simulink model "bipedal_robot_buV2_4"  (R2020b)
settings: Solver=ode23  StartTime=0.0  StopTime=Tsim  MaxStep=0.01  RelTol=1e-3  AbsTol=1e-3  EnableMultiTasking=on
undefined symbols (not defined in the file): Base, ctrl_config, ctrl_data, g, LefAnklePitch, LefAnkleRoll, LefHipPitch, LefHipRoll, LefHipYaw, LefKnee, lleg_str, RigAnklePitch, RigAnkleRoll, RigHipPitch, RigHipRoll, RigHipYaw, RigKnee, rleg_str, sim_floor, Tfil, TG_test_type, total_mass, Ts, X, Y, Z
libraries: sm_lib x53, biped_lib x34, nesl_utility x9, robotmaniplib x5, simulink x1, Contact_Forces_Lib x1
(part 3 of 3)

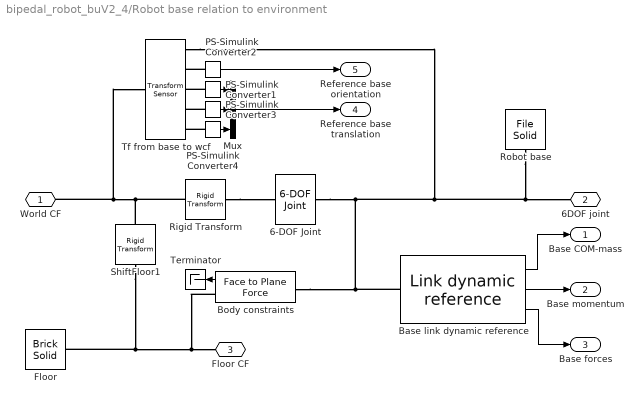
== system bipedal_robot_buV2_4/Robot base relation to environment ==
  6-DOF Joint : sm_lib/Joints/6-DOF Joint  JointMode=Normal  SenseConstraintForce=off  SenseConstraintForceX=off  SenseConstraintForceY=off  SenseConstraintForceZ=off  SenseConstraintTorque=off  SenseConstraintTorqueX=off  SenseConstraintTorqueY=off  SenseConstraintTorqueZ=off  SenseTotalForce=off  SenseTotalForceX=off  SenseTotalForceY=off  SenseTotalForceZ=off  SenseTotalTorque=off  SenseTotalTorqueX=off  SenseTotalTorqueY=off  SenseTotalTorqueZ=off  CompositeWrenchDir=FollowerOnBase  CompositeWrenchFrame=BaseFrame  PxEquilibriumPosition=0  PxEquilibriumPositionUnits=m  PxSpringStiffness=0  PxSpringStiffnessUnits=N/m  PxDampingCoefficient=0  PxDampingCoefficientUnits=N/(m/s)  PxTorqueActuationMode=NoTorque  PxMotionActuationMode=ComputedMotion  PxSensePosition=off  PxSenseVelocity=off  PxSenseAcceleration=off  PxSenseTorqueForce=off  PxSenseLowerLimitTorqueForce=off  PxSenseUpperLimitTorqueForce=off  PxLowerLimitSpecify=off  PxLowerLimitBound=-1  PxLowerLimitBoundUnits=m  PxLowerLimitStiffness=1e6  PxLowerLimitStiffnessUnits=N/m  PxLowerLimitDamping=1e3  PxLowerLimitDampingUnits=N/(m/s)  PxLowerLimitTransitionRegionWidth=1e-4  PxLowerLimitTransitionRegionWidthUnits=m  PxUpperLimitSpecify=off  PxUpperLimitBound=1  PxUpperLimitBoundUnits=m  PxUpperLimitStiffness=1e6  PxUpperLimitStiffnessUnits=N/m  PxUpperLimitDamping=1e3  PxUpperLimitDampingUnits=N/(m/s)  PxUpperLimitTransitionRegionWidth=1e-4  PxUpperLimitTransitionRegionWidthUnits=m  PxPositionTargetSpecify=on  PxPositionTargetPriority=High  PxPositionTargetValue=Base.Xinit(1)  PxPositionTargetValueUnits=m  PxVelocityTargetSpecify=off  PxVelocityTargetPriority=High  PxVelocityTargetValue=0  PxVelocityTargetValueUnits=m/s  PyEquilibriumPosition=0  PyEquilibriumPositionUnits=m  PySpringStiffness=0  PySpringStiffnessUnits=N/m  PyDampingCoefficient=0  PyDampingCoefficientUnits=N/(m/s)  PyTorqueActuationMode=NoTorque  PyMotionActuationMode=ComputedMotion  PySensePosition=off  PySenseVelocity=off  PySenseAcceleration=off  PySenseTorqueForce=off  PySenseLowerLimitTorqueForce=off  PySenseUpperLimitTorqueForce=off  PyLowerLimitSpecify=off  PyLowerLimitBound=-1  PyLowerLimitBoundUnits=m  PyLowerLimitStiffness=1e6  PyLowerLimitStiffnessUnits=N/m  PyLowerLimitDamping=1e3  PyLowerLimitDampingUnits=N/(m/s)  PyLowerLimitTransitionRegionWidth=1e-4  PyLowerLimitTransitionRegionWidthUnits=m  PyUpperLimitSpecify=off  PyUpperLimitBound=1  PyUpperLimitBoundUnits=m  PyUpperLimitStiffness=1e6  PyUpperLimitStiffnessUnits=N/m  PyUpperLimitDamping=1e3  PyUpperLimitDampingUnits=N/(m/s)  PyUpperLimitTransitionRegionWidth=1e-4  PyUpperLimitTransitionRegionWidthUnits=m  PyPositionTargetSpecify=on  PyPositionTargetPriority=High  PyPositionTargetValue=Base.Xinit(2)  PyPositionTargetValueUnits=m  PyVelocityTargetSpecify=off  PyVelocityTargetPriority=High  PyVelocityTargetValue=0  PyVelocityTargetValueUnits=m/s  PzEquilibriumPosition=0  PzEquilibriumPositionUnits=m  PzSpringStiffness=0  PzSpringStiffnessUnits=N/m  PzDampingCoefficient=0  PzDampingCoefficientUnits=N/(m/s)  PzTorqueActuationMode=NoTorque  PzMotionActuationMode=ComputedMotion  PzSensePosition=off  PzSenseVelocity=off  PzSenseAcceleration=off  PzSenseTorqueForce=off  PzSenseLowerLimitTorqueForce=off  PzSenseUpperLimitTorqueForce=off  PzLowerLimitSpecify=off  PzLowerLimitBound=0  PzLowerLimitBoundUnits=m  PzLowerLimitStiffness=1e6  PzLowerLimitStiffnessUnits=N/m  PzLowerLimitDamping=1e3  PzLowerLimitDampingUnits=N/(m/s)  PzLowerLimitTransitionRegionWidth=1e-4  PzLowerLimitTransitionRegionWidthUnits=m  PzUpperLimitSpecify=off  PzUpperLimitBound=1  PzUpperLimitBoundUnits=m  PzUpperLimitStiffness=1e6  PzUpperLimitStiffnessUnits=N/m  PzUpperLimitDamping=1e3  PzUpperLimitDampingUnits=N/(m/s)  PzUpperLimitTransitionRegionWidth=1e-4  PzUpperLimitTransitionRegionWidthUnits=m  PzPositionTargetSpecify=on  PzPositionTargetPriority=High  PzPositionTargetValue=Base.Xinit(3)  PzPositionTargetValueUnits=m  PzVelocityTargetSpecify=off  PzVelocityTargetPriority=High  PzVelocityTargetValue=0  PzVelocityTargetValueUnits=m/s  SphDefPosRotationMethod=None  SphDefPosRotationAngleUnits=deg  SphDefPosRotationStandardAxis=+Z  SphDefPosRotationAngle=0.0  SphDefPosRotationArbitraryAxis=[0 0 1]  SphDefPosFollAlignAxisA=+X  SphDefPosBaseAlignAxisA=+Y  SphDefPosFollAlignAxisB=+Y  SphDefPosBaseAlignAxisB=+Z  SphDefPosRotationSequenceAxes=FollowerAxes  SphDefPosRotationSequence=XYX  SphDefPosRotationSequenceAngles=[0 0 0]  SphDefPosRotationSequenceAnglesUnits=deg  SphDefPosRotationMatrix=[1 0 0; 0 1 0; 0 0 1]  SphEqPosRotationMethod=None  SphEqPosRotationAngleUnits=deg  SphEqPosRotationStandardAxis=+Z  SphEqPosRotationAngle=0.0  SphEqPosRotationArbitraryAxis=[0 0 1]  SphEqPosFollAlignAxisA=+X  SphEqPosBaseAlignAxisA=+Y  SphEqPosFollAlignAxisB=+Y  SphEqPosBaseAlignAxisB=+Z  SphEqPosRotationSequenceAxes=FollowerAxes  SphEqPosRotationSequence=XYX  SphEqPosRotationSequenceAngles=[0 0 0]  SphEqPosRotationSequenceAnglesUnits=deg  SphEqPosRotationMatrix=[1 0 0; 0 1 0; 0 0 1]  SphSpringStiffness=0  SphSpringStiffnessUnits=N*m/deg  SphDampingCoefficient=0  SphDampingCoefficientUnits=N*m/(deg/s)  SphActuateTorqueX=off  SphActuateTorqueY=off  SphActuateTorqueZ=off  SphActuateTorque=off  SphTorqueActuationMode=NoTorque  SphMotionActuationMode=ComputedMotion  SphActuationFrame=BaseFrame  SphSensePosition=off  SphSenseVelocityX=off  SphSenseVelocityY=off  SphSenseVelocityZ=off  SphSenseVelocity=off  SphSenseAccelerationX=off  SphSenseAccelerationY=off  SphSenseAccelerationZ=off  SphSenseAcceleration=off  SphSenseTorqueX=off  SphSenseTorqueY=off  SphSenseTorqueZ=off  SphSenseTorqueForce=off  SphSenseLowerLimitTorqueMag=off  SphSenseUpperLimitTorqueMag=off  SphSensingFrame=BaseFrame  SphLowerLimitSpecify=off  SphLowerLimitBound=15  SphLowerLimitBoundUnits=deg  SphLowerLimitStiffness=1e4  SphLowerLimitStiffnessUnits=N*m/deg  SphLowerLimitDamping=10  SphLowerLimitDampingUnits=N*m/(deg/s)  SphLowerLimitTransitionRegionWidth=0.1  SphLowerLimitTransitionRegionWidthUnits=deg  SphUpperLimitSpecify=off  SphUpperLimitBound=45  SphUpperLimitBoundUnits=deg  SphUpperLimitStiffness=1e4  SphUpperLimitStiffnessUnits=N*m/deg  SphUpperLimitDamping=10  SphUpperLimitDampingUnits=N*m/(deg/s)  SphUpperLimitTransitionRegionWidth=0.1  SphUpperLimitTransitionRegionWidthUnits=deg  SphPositionTargetRotationMethod=StandardAxis  SphPositionTargetRotationAngleUnits=rad  SphPositionTargetRotationStandardAxis=+Y  SphPositionTargetRotationAngle=0  SphPositionTargetRotationArbitraryAxis=[0 0 1]  SphPositionTargetFollAlignAxisA=+X  SphPositionTargetBaseAlignAxisA=+Y  SphPositionTargetFollAlignAxisB=+Y  SphPositionTargetBaseAlignAxisB=+Z  SphPositionTargetRotationSequenceAxes=FollowerAxes  SphPositionTargetRotationSequence=XYX  SphPositionTargetRotationSequenceAngles=[0 0 0]  SphPositionTargetRotationSequenceAnglesUnits=deg  SphPositionTargetRotationMatrix=[1 0 0; 0 1 0; 0 0 1]  SphPositionTargetSpecify=on  SphPositionTargetPriority=High  SphVelocityTargetValue=[0 0 0]  SphVelocityTargetValueUnits=deg/s  SphVelocityTargetSpecify=off  SphVelocityTargetPriority=High  SphVelocityTargetInFollowerFrame=on
  Base link dynamic reference : biped_lib/Link dynamic reference  M=Base.body.mass  I=Base.body.inertia
  Body constraints : Contact_Forces_Lib/3D/Composite Forces/Face to Plane Force  PlaB_x=sim_floor.dims(1)  PlaB_y=sim_floor.dims(2)  PlaB_z=sim_floor.dims(3)/2  FacF_x=Base.dims(1)  FacF_y=Base.dims(2)  FacF_z=Base.dims(3)/2  FacF_rSph=0.01  force_law_pla2pla=Linear  k_contact_pla2pla=Kcont  b_contact_pla2pla=Dcont  pen_full_damp_F_pla2pla=1e-4  pen_exponent_pla2pla=1  friction_law_pla2pla=Stick-Slip Continuous  mu_kinetic_pla2pla=0.5  mu_static_pla2pla=0.7  v_thr_pla2pla=0.001  vis_on_pla2pla=off  vis_opc_en_box2box=0  vis_len_plaLz=0.005  vis_clr=[0.9 0.2 0.2]  vis_opc=0.7
      settings: SourceProductName=Simscape Multibody Contact Forces Library
  Floor : sm_lib/Body Elements/Brick Solid  GraphicAmbientColor=[0.15 0.15 0.15 1.0]  BasedOnType=Density  BrickDimensions=sim_floor.dims  BrickDimensionUnits=m  CenterOfMass=[0 0 0]  CenterOfMassUnits=m  GraphicDiffuseColor=[0.8 0.8 0.8]  Density=1000  DensityUnits=kg/m^3  DoExposeReferenceFrame=on  GraphicEmissiveColor=[0.0 0.0 0.0 1.0]  ExportEntireGeometry=off  SerializedFrames=<Frames/>  MarkerShape=Sphere  MarkerSize=10  GraphicType=FromGeometry  InertiaType=CalculateFromGeometry  Mass=1  MassUnits=kg  MomentsOfInertia=[1 1 1]  MomentsOfInertiaUnits=kg*m^2  GraphicOpacity=1.0  ProductsOfInertia=[0 0 0]  ProductsOfInertiaUnits=kg*m^2  GraphicShininess=75  GraphicSpecularColor=[0.5 0.5 0.5 1.0]  GraphicVisPropType=SimpleVisualProperties
      settings: SourceProductName=Multibody
  Mux : Mux  Inputs=3
  PS-Simulink Converter{1..4} (4 alike) : nesl_utility/PS-Simulink Converter  PhysicalDomain=network_engine_domain  SubClassName=ps_output  LeftPortType=input  RightPortType=output  PseudoPeriodic=off  Frequencies=[]  Unit=1  AffineConversion=off
  Rigid Transform : sm_lib/Frames and Transforms/Rigid Transform  TranslationMethod=StandardAxis  TranslationStandardOffset=0  TranslationLengthUnit=m  TranslationStandardAxis=+Z  TranslationCartesianOffset=[0 0 0]  TranslationROffset=0  TranslationROffsetUnits=m  TranslationZOffset=0  TranslationZOffsetUnits=m  TranslationThetaOffset=0  TranslationThetaOffsetUnits=deg  RotationMethod=None  RotationAngleUnits=deg  RotationStandardAxis=+Z  RotationAngle=0.0  RotationArbitraryAxis=[0 0 1]  FollAlignAxisA=+X  BaseAlignAxisA=+Y  FollAlignAxisB=+Y  BaseAlignAxisB=+Z  RotationSequenceAxes=FollowerAxes  RotationSequence=XYX  RotationSequenceAngles=[0 0 0]  RotationSequenceAnglesUnits=deg  RotationMatrix=[1 0 0; 0 1 0; 0 0 1]
  Robot base : sm_lib/Body Elements/File Solid  ExtGeomFileName=Base_LR.stl  UnitType=Custom  ExtGeomFileUnits=mm  StepReaderType=HEX  ExportConvexHullGeometry=on  InertiaType=CalculateFromGeometry  Mass=Base.body.mass  MassUnits=kg  CenterOfMass=[0 0 0]  CenterOfMassUnits=m  MomentsOfInertia=[1 1 1]  MomentsOfInertiaUnits=kg*m^2  ProductsOfInertia=[0 0 0]  ProductsOfInertiaUnits=kg*m^2  BasedOnType=Mass  Density=1000  DensityUnits=kg/m^3  DoExposeReferenceFrame=on  SerializedFrames=<Frames/>  GraphicType=FromGeometry  MarkerShape=Sphere  MarkerSize=10  GraphicVisPropType=SimpleVisualProperties  GraphicDiffuseColor=[0.5 0.5 0.5]  GraphicSpecularColor=[0.5 0.5 0.5 1.0]  GraphicAmbientColor=[0.15 0.15 0.15 1.0]  GraphicEmissiveColor=[0.0 0.0 0.0 1.0]  GraphicShininess=75  GraphicOpacity=1.0
  ShiftFloor1 : sm_lib/Frames and Transforms/Rigid Transform  TranslationMethod=StandardAxis  TranslationStandardOffset=-sim_floor.dims(3)/2  TranslationLengthUnit=m  TranslationStandardAxis=+Z  TranslationCartesianOffset=[0 0 0]  TranslationROffset=0  TranslationROffsetUnits=m  TranslationZOffset=0  TranslationZOffsetUnits=m  TranslationThetaOffset=0  TranslationThetaOffsetUnits=deg  RotationMethod=None  RotationAngleUnits=deg  RotationStandardAxis=+Z  RotationAngle=0.0  RotationArbitraryAxis=[0 0 1]  FollAlignAxisA=+X  BaseAlignAxisA=+Y  FollAlignAxisB=+Y  BaseAlignAxisB=+Z  RotationSequenceAxes=FollowerAxes  RotationSequence=XYX  RotationSequenceAngles=[0 0 0]  RotationSequenceAnglesUnits=deg  RotationMatrix=[1 0 0; 0 1 0; 0 0 1]
  Terminator : Terminator
  Tf from base to wcf : sm_lib/Frames and Transforms/Transform Sensor  MeasurementFrame=World  SenseAngle=off  SenseAxis=off  SenseAngle1=off  SenseAngle2=off  SenseAngle3=off  SenseQ=off  SenseR=on  SenseOmegaX=off  SenseOmegaY=off  SenseOmegaZ=off  SenseOmega1=off  SenseOmega2=off  SenseOmega3=off  SenseQDot=off  SenseRDot=off  SenseAlphaX=off  SenseAlphaY=off  SenseAlphaZ=off  SenseAlpha1=off  SenseAlpha2=off  SenseAlpha3=off  SenseQDDot=off  SenseRDDot=off  SenseX=on  SenseY=on  SenseZ=on  SenseRad=off  SenseAzim=off  SenseDist=off  SenseInc=off  SenseXDot=off  SenseYDot=off  SenseZDot=off  SenseRadDot=off  SenseAzimDot=off  SenseDistDot=off  SenseIncDot=off  SenseXDDot=off  SenseYDDot=off  SenseZDDot=off  SenseRadDDot=off  SenseAzimDDot=off  SenseDistDDot=off  SenseIncDDot=off
  World CF : PMIOPort  Side=Left
  6DOF joint : PMIOPort  Port=2  Side=Right
  Floor CF : PMIOPort  Port=3  Side=Right
  Base COM-mass : Outport
  Base momentum : Outport  Port=2
  Base forces : Outport  Port=3
  Reference base translation : Outport  Port=4
  Reference base orientation : Outport  Port=5
  wires:
  Body constraints/1 -> Terminator/1
  Base link dynamic reference/1 -> Base COM-mass/1
  Base link dynamic reference/2 -> Base momentum/1
  Base link dynamic reference/3 -> Base forces/1
  PS-Simulink Converter2/1 -> Reference base orientation/1
  PS-Simulink Converter3/1 -> Mux/2
  PS-Simulink Converter1/1 -> Mux/1
  PS-Simulink Converter4/1 -> Mux/3
  Mux/1 -> Reference base translation/1
  connections:
  Rigid Transform/LConn1 -- Tf from base to wcf/LConn1 -- World CF/RConn1 -- ShiftFloor1/LConn1
  Rigid Transform/RConn1 -- 6-DOF Joint/LConn1
  6-DOF Joint/RConn1 -- Tf from base to wcf/RConn1 -- Robot base/RConn1 -- 6DOF joint/RConn1 -- Base link dynamic reference/LConn1 -- Body constraints/LConn1
  ShiftFloor1/RConn1 -- Floor/RConn1 -- Floor CF/RConn1 -- Body constraints/RConn1
  PS-Simulink Converter2/LConn1 -- Tf from base to wcf/RConn2
  PS-Simulink Converter1/LConn1 -- Tf from base to wcf/RConn3
  PS-Simulink Converter3/LConn1 -- Tf from base to wcf/RConn4
  PS-Simulink Converter4/LConn1 -- Tf from base to wcf/RConn5

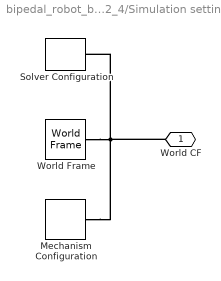
== system bipedal_robot_buV2_4/Simulation settings ==
  Mechanism Configuration : sm_lib/Utilities/Mechanism Configuration  UniformGravity=Constant  GravityVector=gvec  GravityVectorUnits=m/s^2  GravityUnits=m/s^2  LinearizationDelta=0.001  JointModeTransitionNonlinearIterations=2
      settings: SourceProductName=Multibody
  Solver Configuration : nesl_utility/Solver Configuration  PhysicalDomain=network_engine_domain  SubClassName=solver  LeftPortType=input  RightPortType=generic  Tones=[]  Harmonics=[]  SimulateNoise=off  Profile=off  UseLocalSampling=off  EnableSwitchedLinearOptims=on  FrequencyDomain=off  UseCCode=off  RelTol=0.001  AbsTol=1e-06  MinStep=1e-09  ToWorkspace=off  RevertToSquareIcSolve=off  NumHomotopyIterations=100  PhasorMode=off  PhasorModeNumHarmonics=1  DoDC=off  ResidualTolerance=1e-09  UseLocalSolver=off  LocalSolverChoice=NE_BACKWARD_EULER_ADVANCER  LocalSolverSampleTime=0.001  DoFixedCost=off  MaxNonlinIter=3  MaxModeIter=2  ComputeImpulses=off  ImpulseIterations=2  LinearAlgebra=Sparse  EquationFormulation=NE_TIME_EF  DelaysMemoryBudget=1024  AutomaticFiltering=on  FilteringTimeConstant=0.001  PartitionStorageMethod=AS_NEEDED  PartitionMemoryBudget=1024  PartitionMethod=FAST
      settings: SourceProductName=Utilities
  World Frame : sm_lib/Frames and Transforms/World Frame
      settings: SourceProductName=Multibody
  World CF : PMIOPort  Side=Right
  connections:
  World Frame/RConn1 -- World CF/RConn1 -- Solver Configuration/RConn1 -- Mechanism Configuration/RConn1

== matlab function bipedal_robot_buV2_4/Controller/Sensor mapping ==
  data: MSL input; Qconfig output; MSR input
function Qconfig = fcn(MSL,MSR)
    [LL,RL] = group_motor_data(MSL,MSR);
    Qconfig = zeros(12,1);
    %joints start at hip and go down to ankle. Left and right joints are
    %always following one another
    Qconfig(1:2:end) = LL.q;
    Qconfig(2:2:end) = RL.q;
    %if using roby
    %Qconfig(1:end/2) = LL.q;
    %Qconfig(end/2+1:end) = RL.q;

== matlab function bipedal_robot_buV2_4/Controller/Walking controller ==
  data: time input; MSL input; TL output; LFL input; MSR input; LFR input; ZMP_ref input; TR output; COM_des output; p_des output; COM_ref input; ctrl_data input; ctrl_config input; twb input; Rwb input; GenMotion input; p_ref output; p_qp output; dcm_des output; dcm_meas output; test_type input; e_qL output; e_qR output
function [TL,TR, COM_des, p_des, p_ref, p_qp, dcm_des, dcm_meas, e_qL, e_qR] = fcn(time, MSL,LFL,MSR,LFR, ZMP_ref, COM_ref, ctrl_data, ctrl_config, twb, Rwb, GenMotion, test_type)
persistent dcm_int;
persistent init_corr corr_stored;

if isempty(dcm_int)
    dcm_int = zeros(2,1); %initialise the integrator
    corr_stored = zeros(3,1);
end

%% constants & configuration

z_des = ctrl_config.com_height;
g = 9.81;
omega = sqrt(g/z_des);
zp_des = 0;
Mtot = ctrl_config.mass;
foot_dims = ctrl_config.foot_dims*0.7;
K = Mtot*omega^2;

%% values from the pattern generator
if test_type == 0
    %only stabilization (trajectories are not used) => disturbance test
    phase = 0; %DS all the time
    WshiftL = 0.5; %equal wrench distribution
    WshiftR = 0.5;
    ZMP_des = ctrl_config.pdes_ini;
    COM_des = ZMP_des;
    COMp_des = zeros(2,1);
    qL_des = ctrl_config.qLd;
    qR_des = ctrl_config.qRd;
    qLp_des = zeros(6,1);
    qRp_des = zeros(6,1);
else
    % all the other tests require a trajectory
    if test_type == 1
        % shifting the weight only
        phase = 0;  % always remain in DS phase
    else
        % lifting the swing leg
        phase = GenMotion(1);
    end
    WshiftL = GenMotion(2);
    WshiftR = GenMotion(3);
    ZMP_des = GenMotion(4:5);
    COM_des = GenMotion(6:7);
    COMp_des = GenMotion(8:9);
    qL_des = GenMotion(10:15);
    qR_des = GenMotion(16:21);
    qLp_des = GenMotion(22:27);
    qRp_des = GenMotion(28:33);
end

%% Desired state values
%desired joint angles
qLd = qL_des;%qLd = ctrl_config.qLd;
qRd = qR_des;%qRd = ctrl_config.qRd;
%desired joint velocities
qLpd = qLp_des;
qRpd = qRp_des;
% desired ZMP
p_des = ZMP_des; %p_des = ctrl_config.pdes_ini(1:2) + dcm_offs;
% desired COM
C_d = COM_des;%C_d = p_des;zeros(3,1);
Cp_d = COMp_des;%Cp_d = [0,0]';
% desired DCM
dcm_des = C_d + Cp_d/omega;


%% Measurements from motors
[LL,RL] = group_motor_data(MSL,MSR);
qL = LL.q;
qR = RL.q;
qLp = LL.qp;
qRp = RL.qp;

%% COM & ZMP observer (Now: reference data - Todo: implment an observer)
C_meas = COM_ref(1:3);
Cp_meas = COM_ref(4:6);
p_meas = ZMP_ref;


%% COM controller 
% gain setup
sc = omega;
Kp_com = [3.5*sc;5.0*sc];
Kp_comz = 500*sc;
Kd_com = 100*sc;
Kp_p = [0.9*sc;0.2*sc];

% leaky integrator
Ki_com = [1*sc;2*sc];
Kleak = [0.1;0.1];

% control law for COM forces
if C_meas(3)==0
    czerr = 0;
    C_meas_ada = C_meas;
else
    if isempty(init_corr)
        init_corr = 1;
        corr_stored = C_meas - [0;0;z_des];
    end
    C_meas_ada = C_meas - [0,0,corr_stored(3)]'; %this will have to be performed in practice as well
    %C_meas_ada = C_meas - corr_stored;
    
    czerr = Kd_com*(zp_des - Cp_meas(3)) + Kp_comz*(z_des-C_meas_ada(3));
end

%% DCM observer
dcm_meas = C_meas_ada(1:2) + C_meas_ada(1:2)/omega;
% integrate the DCM error (IIR filter)
dT = 1/ctrl_config.fctrl;
dcm_err = dcm_des - dcm_meas; %integral error
d_err = dcm_err - Kleak.*dcm_int; %inclusion of leakage
dcm_int = dcm_int + dT * d_err;

%% CONTROLLER
% reference value for the ZMP
p_ref = p_des -(1+Kp_com./omega).*dcm_err - Ki_com./omega.*dcm_int + Kp_p./omega.*(p_des-p_meas);

Fd = [
    -K*(C_meas_ada(1)-p_ref(1));
    -K*(C_meas_ada(2)-p_ref(2));
    -(Mtot*g + czerr);
];

% control law for torques around COM
% angular velocities measured in motors attached rigidly to base (M1 - L&R)
%left measurement
w_1L = LL.w(:,1);
R_base_IMU_1L = rotz(-pi/6);
wbaseL = R_base_IMU_1L*w_1L;
%right measurement
w_1R = RL.w(:,1);
R_base_IMU_1R = rotz(+pi/6);
wbaseR = R_base_IMU_1R*w_1R;
%average both
omega=(wbaseL+wbaseR)/2;
Td = floating_base_orientation(Rwb',omega); %transpose the rotm to get the correct mapping (FROM:desired TO:actual)
%Td = zeros(3,1);
% generate an overall wrench (in the world frame)
Wc = [Fd;Td]; 

% get jaccobians 
% WATCH OUT => First lines 1-3 are Jw and 4-6 are Jv (swapped rot. and tr.
% motion)
JL = ctrl_data.JL(:,1:2:end); 
JLcorr = [JL(4:6,:);JL(1:3,:)];

JR = ctrl_data.JR(:,2:2:end);
JRcorr = [JR(4:6,:);JR(1:3,:)];

% get transformations (feet to base)
TF_world_base = [
    Rwb, twb;
    zeros(1,3),1
];

TF_world_com = [
    eye(3),C_meas;
    zeros(1,3),1
];

TF_com_base = TF_world_com\TF_world_base; %TF from base to COM

TF_eeL_base = ctrl_data.TL; %TF from left end effector to base
TF_eeR_base = ctrl_data.TR; %TF from right end effector to base

% get required wrench mappings
AdT_gcb = Ad_g(TF_com_base(1:3,1:3),TF_com_base(1:3,4))';
AdT_gbl = Ad_g(TF_eeL_base(1:3,1:3),TF_eeL_base(1:3,4))';
AdT_gbr = Ad_g(TF_eeR_base(1:3,1:3),TF_eeR_base(1:3,4))';

%% torque distribution
% transform the wrench from com to the body frame (gcb transforms vectors
% from base to com, but AdT is dual - transforms in the oposite order)
%Wb = AdT_gcb*Wc;
% equally distribute the wrench and transform them to the feet frames
%Wlfoot = AdT_gbl*Wb /2;
%Wrfoot = AdT_gbr*Wb /2;
[Wlfoot,Wrfoot] = distribute_wrench_tracking(Wc,JLcorr,JRcorr,TF_com_base,TF_eeL_base,TF_eeR_base,foot_dims,0.6,0,phase,WshiftL,WshiftR);
% map the wrenches to respective joint torques
TLtc = JLcorr'*Wlfoot;
TRtc = JRcorr'*Wrfoot;


%% Test if the zmp recomputation matters
TF_world_eeL = TF_world_base*inv(TF_eeL_base);
TF_world_eeR = TF_world_base*inv(TF_eeR_base);
RwL = TF_world_eeL(1:3,1:3);
RwR = TF_world_eeR(1:3,1:3);
twL = TF_world_eeL(1:3,4);
twR = TF_world_eeR(1:3,4);
[pL,Wlfoot_rot] = zmp_from_wrench(Wlfoot,RwL,twL);
[pR,Wrfoot_rot] = zmp_from_wrench(Wrfoot,RwR,twR);
p_qp = (Wlfoot_rot(3)*pL+Wrfoot_rot(3)*pR)/(Wlfoot_rot(3)+Wrfoot_rot(3));

%% Joint control (secondary task)
[KpL, KpR, KdL, KdR] = get_gains(test_type, phase, WshiftL, WshiftR);

% compute errors
e_qL = qLd-qL;
e_qR = qRd-qR;
ep_qL = qLpd-qLp;
ep_qR = qRpd-qRp;
% separated pd control
TLpos = KpL.*e_qL;
TRpos = KpR.*e_qR;
TLvel = KdL.*ep_qL;
TRvel = KdR.*ep_qR;

% Null space projector (for a 2 level hierarchy, successive and augmented projectors are the same)
use_NS_ctrl = 2;
if use_NS_ctrl && phase == 0 %can only be used in DS phase
    rho = 0.1; %needs to be included
    Jfull = [JLcorr,JRcorr];
    JLpseud = pseudoinv(Jfull,rho,'right');
    % compute the projector
    Nproj2 = (eye(12)-Jfull'*JLpseud');
    % project the secondary task to the nullspace of the primary one
    if use_NS_ctrl==1
        %only position is projected 
        Tsec = Nproj2*[TLpos;TRpos];
        TLsec = Tsec(1:end/2);
        TRsec = Tsec(end/2+1:end);
        %velocity is added
        TLsec = TLsec + TLvel;
        TRsec = TRsec + TLvel;
    elseif use_NS_ctrl==2
        %position and velocity are projected
        Tsec = Nproj2*[TLpos+TLvel;TRpos+TRvel];
        TLsec = Tsec(1:end/2);
        TRsec = Tsec(end/2+1:end);
    end
else
    % simply add the secondary task to the primary on
    TLsec = TLpos + TLvel;
    TRsec = TRpos + TLvel;
    if phase == 1
        Grem = rtbox_to_alg(ctrl_data.G);
        Gl = Grem(1:end/2);
        Gr = Grem(end/2+1:end);
        if WshiftL>WshiftR
            %right leg is swinging
            TRsec = TRsec + Gr;
        else
            %left leg is swinging
            TLsec = TLsec + Gl;
        end
    end
end


    

%% Combined control
TL = TLtc + TLsec;
TR = TRtc + TRsec;
